simulink model "simulink_control"  (R2024b)
settings: Solver=ode5  StartTime=0.0  StopTime=inf  FixedStep=0.016  RelTol=1e-3
values from neighbouring files (symbols this model uses):
  gps = wb_robot_get_device('gps')    [crazyflie_simulink_control.m]
  gyro = wb_robot_get_device('gyro')    [crazyflie_simulink_control.m]
  imu = wb_robot_get_device('inertial unit')    [crazyflie_simulink_control.m]
  m1_motor = wb_robot_get_device('m1_motor')    [crazyflie_simulink_control.m]
  m2_motor = wb_robot_get_device('m2_motor')    [crazyflie_simulink_control.m]
  m3_motor = wb_robot_get_device('m3_motor')    [crazyflie_simulink_control.m]
  m4_motor = wb_robot_get_device('m4_motor')    [crazyflie_simulink_control.m]
  range_back = wb_robot_get_device('range_back')    [crazyflie_simulink_control.m]
  range_front = wb_robot_get_device('range_front')    [crazyflie_simulink_control.m]
  range_left = wb_robot_get_device('range_left')    [crazyflie_simulink_control.m]
  range_right = wb_robot_get_device('range_right')    [crazyflie_simulink_control.m]
  TIME_STEP = 16    [crazyflie_simulink_control.m]
undefined symbols (not defined in the file or in its folder): a1, a2, a3, a4, accelerometer_sensor
libraries: eeGeneralControl x1, slpidlib x1
settings Model: Creator=Harun  LastModifiedBy=harunkurtdev

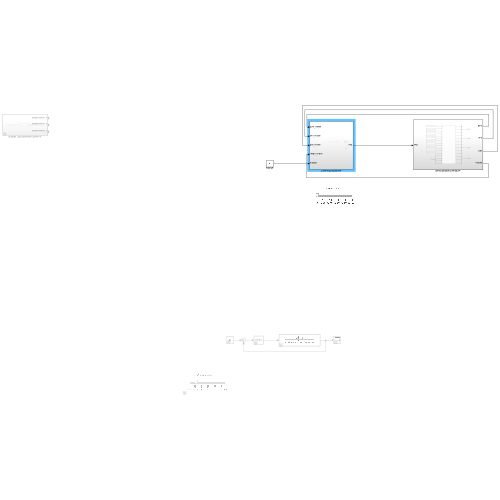
[thumbnail: Simulink's stored preview of the top-level diagram]
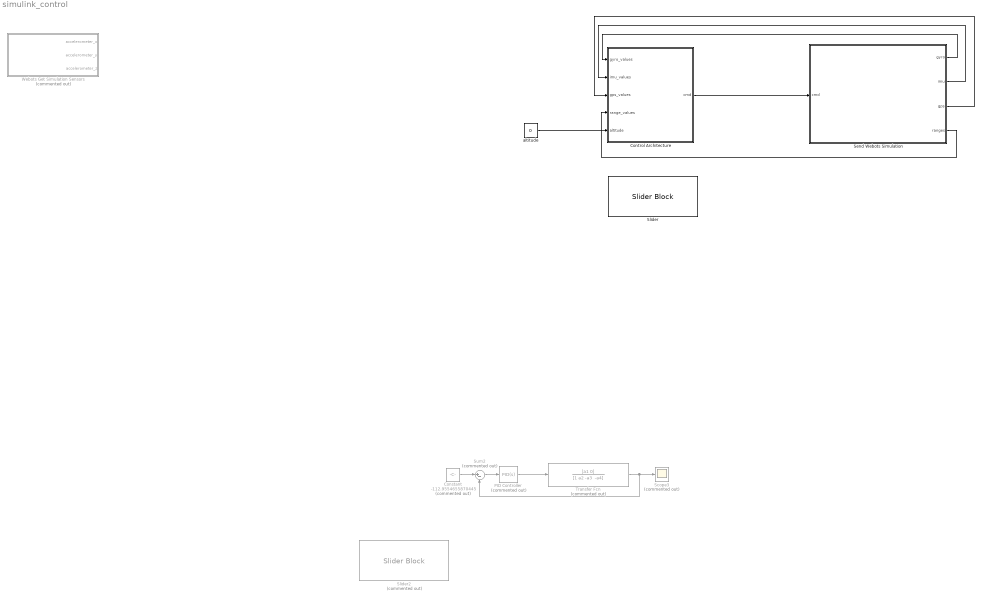
== system simulink_control ==
  Constant : Constant  Commented=on  Value=-112.9554655870445
  Control Architecture : Subsystem
  PID Controller : slpidlib/PID Controller  Commented=on  Controller=PID  Form=Parallel  TimeDomain=Continuous-time  UseExternalTs=off  SampleTime=-1  IntegratorMethod=Forward Euler  FilterMethod=Forward Euler  ControllerParametersSource=internal  P=117.155618821838  I=67.2944879318419  UseKiTs=off  D=44.7801205202101  UseExternalDerivativeSource=off  N=97.4887289682428  UseFilter=on  TunerSelectOption=Transfer Function Based (PID Tuner App)  InitialConditionSource=internal  InitialConditionForIntegrator=0  InitialConditionForFilter=0  DifferentiatorICPrevScaledInput=0  ExternalReset=none  TrackingMode=off  Kt=1  LimitOutput=off  SatLimitsSource=internal  UpperSaturationLimit=inf  LowerSaturationLimit=-inf  LinearizeAsGain=on  AntiWindupMode=none  Kb=1  LimitIntegrator=off  UpperIntegratorSaturationLimit=inf  LowerIntegratorSaturationLimit=-inf  POutMin=[]  POutMax=[]  IOutMin=[]  IOutMax=[]  DOutMin=[]  DOutMax=[]  NOutMin=[]  NOutMax=[]  SumOutMin=[]  SumOutMax=[]  SaturationOutMin=[]  SaturationOutMax=[]  PParamMin=[]  PParamMax=[]  IParamMin=[]  IParamMax=[]  DParamMin=[]  DParamMax=[]  NParamMin=[]  NParamMax=[]  KbParamMin=[]  KbParamMax=[]  KtParamMin=[]  KtParamMax=[]  KbOutMin=[]  KbOutMax=[]  KtOutMin=[]  KtOutMax=[]  IntegratorOutMin=[]  IntegratorOutMax=[]  FilterOutMin=[]  FilterOutMax=[]  SumI1OutMin=[]  SumI1OutMax=[]  SumI2OutMin=[]  SumI2OutMax=[]  SumI3OutMin=[]  SumI3OutMax=[]  SumI4OutMin=[]  SumI4OutMax=[]  SumDOutMin=[]  SumDOutMax=[]  DifferentiatorOutMin=[]  DifferentiatorOutMax=[]  FilterDiffOutCoefMin=[]  FilterDiffOutCoefMax=[]  ReciprocalOutMin=[]  ReciprocalOutMax=[]  SumDenOutMin=[]  SumDenOutMax=[]  SumNumOutMin=[]  SumNumOutMax=[]  DivideOutMin=[]  DivideOutMax=[]  UdiffTsProdOutMin=[]  UdiffTsProdOutMax=[]  NTsProdOutMin=[]  NTsProdOutMax=[]  UintegralTsProdOutMin=[]  UintegralTsProdOutMax=[]  UngainTsProdOutMin=[]  UngainTsProdOutMax=[]  ClampingZeroOutDataTypeStr=Inherit: Inherit via back propagation  ClampingZeroOutMin=[]  ClampingZeroOutMax=[]  FilterDenConstantOutDataTypeStr=Inherit: Inherit via back propagation  FilterDenConstantOutMin=[]  FilterDenConstantOutMax=[]  PCopyOutDataTypeStr=Inherit: Inherit via back propagation  PCopyOutMin=[]  PCopyOutMax=[]  NCopyOutDataTypeStr=Inherit: Inherit via back propagation  NCopyOutMin=[]  NCopyOutMax=[]  IntegratorContinuousStateAttributes=''  IntegratorStateMustResolveToSignalObject=off  IntegratorRTWStateStorageClass=Auto  FilterContinuousStateAttributes=''  FilterStateMustResolveToSignalObject=off  FilterRTWStateStorageClass=Auto  ParallelPVariant=InternalParameters  IdealPVariant=Disabled  IVariant=InternalParameters  DVariant=InternalParameters  IntegratorVariant=Continuous  SatVariant=Disabled  AWVariant=Passthrough  PCopyVariant=Disabled  TRVariant=Disabled  FdbkBlocksVariant=Forward  IdealPFdbkVariant=Disabled  SatFdbkVariant=Disabled  DerivativeFilterVariant=ContFilter  NVariant=InternalParameters  NCopyVariant=Disabled  FilterICVariant=InternalICsFilter  IntegratorICVariant=InternalICs  ExternalResetVariant=Disabled  TRSumVariant=Passthrough  SumFdbkVariant=Disabled  SumVariant=Sum_PID  TsampFilterVariant=InternalTs  TsampNgainVariant=Passthrough  TsampIntegralVariant=Passthrough  ExternalSaturationOutDataTypeStr=Inherit: Same as second input  DerivativeSourceVariant=ErrorSignal  PreIntVariant=InternalPreInt
  Scope3 : Scope  Commented=on
  Send Webots Simulation : Subsystem
  Slider : SliderBlock
  Slider2 : SliderBlock  Commented=on  ScaleMin=-180  ScaleMax=180
  Sum2 : Sum  Commented=on  Inputs=|+-
  Transfer Fcn : TransferFcn  Commented=on  Numerator=[a1 0]  Denominator="[1 a2 -a3  -a4]"
  Webots Get Simulation Sensors : Subsystem  Commented=on
  altitude : Constant  Value=0
  wires:
  PID Controller/1 -> Transfer Fcn/1
  Sum2/1 -> PID Controller/1
  Constant/1 -> Sum2/1
  Transfer Fcn/1 -> Scope3/1, Sum2/2
  Control Architecture/1(cmd) -> Send Webots Simulation/1(cmd)
  Send Webots Simulation/1(gyro) -> Control Architecture/1(gyro_values)
  Send Webots Simulation/2(imu) -> Control Architecture/2(imu_values)
  Send Webots Simulation/3(gps) -> Control Architecture/3(gps_values)
  altitude/1 -> Control Architecture/5(altitude)
  Send Webots Simulation/4(ranges) -> Control Architecture/4(range_values)

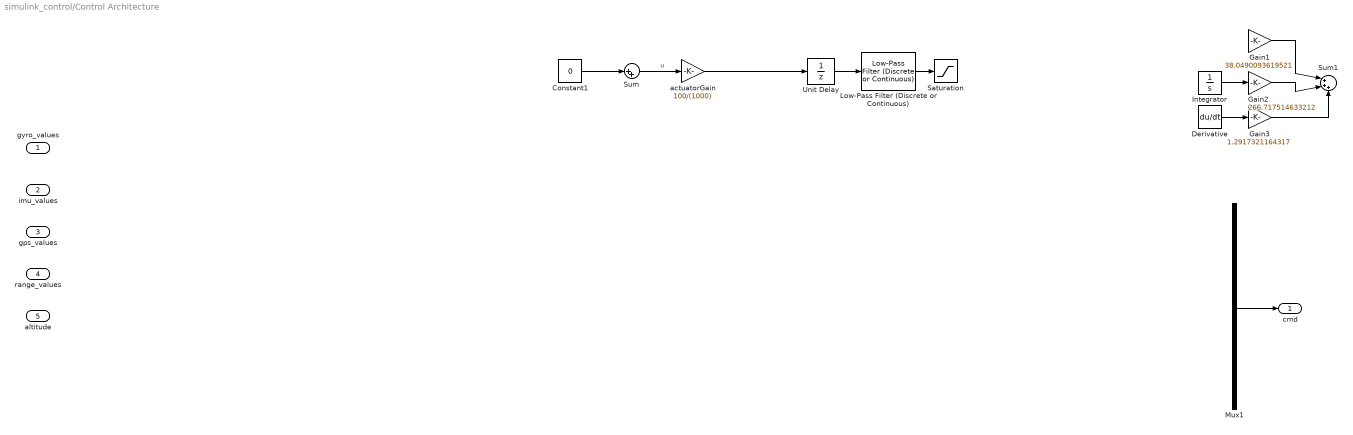
== system simulink_control/Control Architecture ==
  gyro_values : Inport
  imu_values : Inport  Port=2
  gps_values : Inport  Port=3
  range_values : Inport  Port=4
  altitude : Inport  Port=5
  Constant1 : Constant  Value=0
  Derivative : Derivative  CoefficientInTFapproximation=0.016
  Gain1 : Gain  Gain=38.0490093619521
  Gain2 : Gain  Gain=266.717514633212
  Gain3 : Gain  Gain=1.2917321164317
  Integrator : Integrator  AbsoluteTolerance=0.016
  Low-Pass Filter (Discrete or Continuous) : eeGeneralControl/Low-Pass Filter (Discrete or Continuous)  K=1  T=0.016  B=inf  A=-inf  init_option=Inherited from block input  x0=0  Ts=-1
  Mux1 : Mux
  Saturation : Saturate  UpperLimit=100  LowerLimit=-100
  Sum : Sum  Inputs=|++
  Sum1 : Sum  Inputs=|+++
  Unit Delay : UnitDelay  SampleTime=-1  HasFrameUpgradeWarning=on
  actuatorGain : Gain  Gain=100/(1000)
  cmd : Outport
  wires:
  Constant1/1 -> Sum/1
  Sum/1 -> actuatorGain/1  "u"
  Unit Delay/1 -> Low-Pass Filter (Discrete or Continuous)/1
  Low-Pass Filter (Discrete or Continuous)/1 -> Saturation/1
  actuatorGain/1 -> Unit Delay/1
  Mux1/1 -> cmd/1
  Derivative/1 -> Gain3/1
  Integrator/1 -> Gain2/1
  Gain3/1 -> Sum1/3
  Gain1/1 -> Sum1/1
  ? -> Gain1/1, Derivative/1, Integrator/1
  Gain2/1 -> Sum1/2

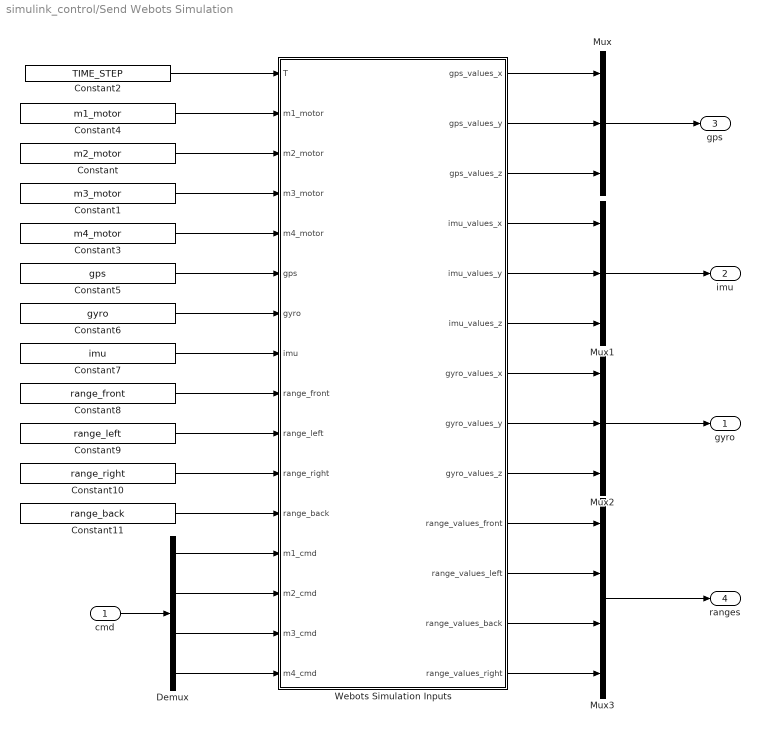
== system simulink_control/Send Webots Simulation ==
  cmd : Inport
  Constant : Constant  Value=m2_motor
  Constant1 : Constant  Value=m3_motor
  Constant10 : Constant  Value=range_right
  Constant11 : Constant  Value=range_back
  Constant2 : Constant  Value=TIME_STEP
  Constant3 : Constant  Value=m4_motor
  Constant4 : Constant  Value=m1_motor
  Constant5 : Constant  Value=gps
  Constant6 : Constant  Value=gyro
  Constant7 : Constant  Value=imu
  Constant8 : Constant  Value=range_front
  Constant9 : Constant  Value=range_left
  Demux : Demux
  Mux : Mux  Inputs=3
  Mux1 : Mux  Inputs=3
  Mux2 : Mux  Inputs=3
  Mux3 : Mux
  Webots Simulation Inputs : MATLAB Function  TreatAsAtomicUnit=on
  gyro : Outport
  imu : Outport  Port=2
  gps : Outport  Port=3
  ranges : Outport  Port=4
  wires:
  Constant2/1 -> Webots Simulation Inputs/1(T)
  Constant4/1 -> Webots Simulation Inputs/2(m1_motor)
  Constant/1 -> Webots Simulation Inputs/3(m2_motor)
  Constant11/1 -> Webots Simulation Inputs/12(range_back)
  Constant10/1 -> Webots Simulation Inputs/11(range_right)
  Constant1/1 -> Webots Simulation Inputs/4(m3_motor)
  Constant3/1 -> Webots Simulation Inputs/5(m4_motor)
  Constant5/1 -> Webots Simulation Inputs/6(gps)
  Constant6/1 -> Webots Simulation Inputs/7(gyro)
  Constant7/1 -> Webots Simulation Inputs/8(imu)
  Constant8/1 -> Webots Simulation Inputs/9(range_front)
  Constant9/1 -> Webots Simulation Inputs/10(range_left)
  Demux/3 -> Webots Simulation Inputs/15(m3_cmd)
  Demux/4 -> Webots Simulation Inputs/16(m4_cmd)
  Demux/2 -> Webots Simulation Inputs/14(m2_cmd)
  Demux/1 -> Webots Simulation Inputs/13(m1_cmd)
  cmd/1 -> Demux/1
  Webots Simulation Inputs/2(gps_values_y) -> Mux/2
  Webots Simulation Inputs/1(gps_values_x) -> Mux/1
  Webots Simulation Inputs/3(gps_values_z) -> Mux/3
  Mux/1 -> gps/1
  Webots Simulation Inputs/5(imu_values_y) -> Mux1/2
  Webots Simulation Inputs/4(imu_values_x) -> Mux1/1
  Webots Simulation Inputs/6(imu_values_z) -> Mux1/3
  Webots Simulation Inputs/7(gyro_values_x) -> Mux2/1
  Webots Simulation Inputs/9(gyro_values_z) -> Mux2/3
  Webots Simulation Inputs/8(gyro_values_y) -> Mux2/2
  Mux1/1 -> imu/1
  Mux2/1 -> gyro/1
  Webots Simulation Inputs/10(range_values_front) -> Mux3/1
  Webots Simulation Inputs/11(range_values_left) -> Mux3/2
  Webots Simulation Inputs/12(range_values_back) -> Mux3/3
  Webots Simulation Inputs/13(range_values_right) -> Mux3/4
  Mux3/1 -> ranges/1

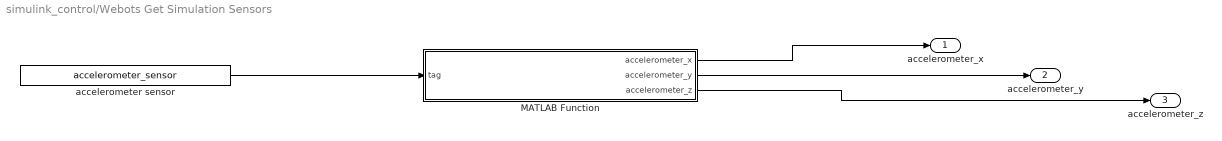
== system simulink_control/Webots Get Simulation Sensors ==
  MATLAB Function : MATLAB Function  TreatAsAtomicUnit=on
  accelerometer sensor : Constant  Value=accelerometer_sensor
  accelerometer_x : Outport
  accelerometer_y : Outport  Port=2
  accelerometer_z : Outport  Port=3
  wires:
  accelerometer sensor/1 -> MATLAB Function/1(tag)
  MATLAB Function/1(accelerometer_x) -> accelerometer_x/1
  MATLAB Function/3(accelerometer_z) -> accelerometer_z/1
  MATLAB Function/2(accelerometer_y) -> accelerometer_y/1

== matlab function simulink_control/Webots Get Simulation Sensors/MATLAB Function ==
  data: tag input; accelerometer_x output; accelerometer_y output; accelerometer_z output
function [accelerometer_x,accelerometer_y,accelerometer_z] = accelerometer_sensor_get(tag)

period = wb_accelerometer_get_sampling_period(tag)
values = wb_accelerometer_get_values(tag);
accelerometer_x = values(1);
accelerometer_y = values(2);
accelerometer_z = values(3);

== matlab function simulink_control/Send Webots Simulation/Webots Simulation Inputs ==
  data: T input; m1_motor input; m2_motor input; m3_motor input; m4_motor input; gps_values_x output; gps_values_y output; gps input; gyro input; imu input; range_front input; range_left input; range_right input; range_back input; m1_cmd input; m2_cmd input; m3_cmd input; m4_cmd input; gps_values_z output; imu_values_x output; imu_values_y output; imu_values_z output; gyro_values_x output; gyro_values_y output; gyro_values_z output; range_values_front output; range_values_left output; range_values_back output; range_values_right output
function [gps_values_x,gps_values_y,gps_values_z,imu_values_x,imu_values_y,imu_values_z,gyro_values_x,gyro_values_y,gyro_values_z,range_values_front,range_values_left,range_values_back,range_values_right]  =   simulation(T,m1_motor,m2_motor,m3_motor,m4_motor,gps,gyro,imu,range_front,range_left,range_right,range_back,m1_cmd,m2_cmd,m3_cmd,m4_cmd)


gps_values=zeros(1,3);
gyro_values=zeros(1,3);
imu_values=zeros(1,3);
range_values=zeros(1,3);

wb_robot_step(T)

imu_values=wb_inertial_unit_get_roll_pitch_yaw(imu);
imu_values_x=imu_values(1);
imu_values_y=imu_values(2);
imu_values_z=imu_values(3);

gyro_values=wb_gyro_get_values(gyro);
gyro_values_x=gyro_values(1);
gyro_values_y=gyro_values(2);
gyro_values_z=gyro_values(3);

gps_values=wb_gps_get_values(gps);
gps_values_x=gps_values(1);
gps_values_y=gps_values(2);
gps_values_z=gps_values(3);

range_values_front=0.0;
range_values_left=0.0;
range_values_right=0.0;
range_values_back=0.0;

wb_motor_set_velocity(m1_motor,-m1_cmd);
wb_motor_set_position(m1_motor,Inf);

wb_motor_set_velocity(m2_motor,m2_cmd);
wb_motor_set_position(m2_motor,Inf);

wb_motor_set_velocity(m3_motor,-m3_cmd);
wb_motor_set_position(m3_motor,Inf);

wb_motor_set_velocity(m4_motor,m4_cmd);
wb_motor_set_position(m4_motor,Inf);


end
